simulink model "robotController"  (R2019b)
settings: Solver=FixedStepAuto  StartTime=0.0  StopTime=10.0  FixedStep=0.1  RelTol=1e-3
InitFcn:
  | set_param('robotController', 'ForceConsistencyChecking', 'off');
undefined symbols (not defined in the file): awayFromGoalThresh, loadingStation, logicalMap, unloadingStations
libraries: robotalgslib x1
settings Model: OrderedModelArguments=off  Creator=The MathWorks, Inc.  LastModifiedBy=Helsi
settings RTWCC: GenCodeOnly=on

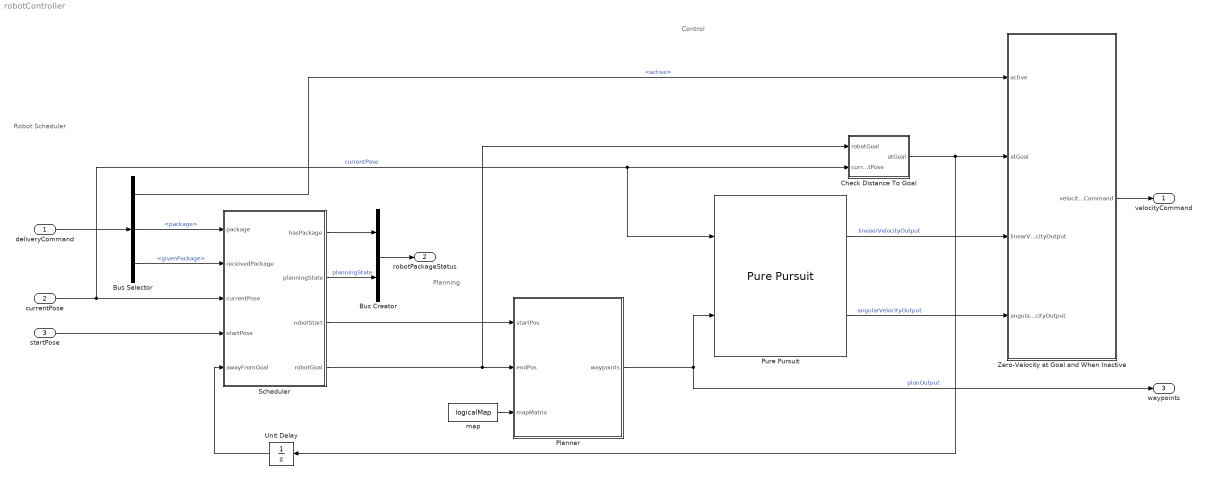
== system robotController ==
  note: Control
  note: Planning
  note: Robot Scheduler
  deliveryCommand : Inport  OutDataTypeStr=Bus: RobotDeliverCommand  BusOutputAsStruct=on
  currentPose : Inport  Port=2  PortDimensions=[3, 1]
  startPose : Inport  Port=3
  Bus Creator : BusCreator  Inputs=2  OutDataTypeStr=Bus: RobotPackageStatus  NonVirtualBus=on
      settings: InheritFromInputs=off
  Bus Selector : BusSelector  OutputSignals=active,package,givenPackage
  Check Distance To Goal : Subsystem
  Planner : MATLAB Function  TreatAsAtomicUnit=on
  Pure Pursuit : robotalgslib/Pure Pursuit  DesiredLinearVelocity=0.1  MaxAngularVelocity=1.0  LookaheadDistance=0.5  TargetDirPort=off  SimulateUsing=Code generation
      settings: SourceProductName=Navigation Toolbox  SourceProductBaseCode=NV
  Scheduler : Stateflow chart  Priority=2  BlockKeywords=__PRM__SERIALIZED__DATA__:Stateflow Chart,Stateflow Diagram
  Unit Delay : UnitDelay  SampleTime=-1  HasFrameUpgradeWarning=on
  Zero-Velocity at Goal and When Inactive : Subsystem
  map : Constant  Value=logicalMap
  velocityCommand : Outport
  robotPackageStatus : Outport  Port=2  OutDataTypeStr=Bus: RobotPackageStatus  BusOutputAsStruct=on
  waypoints : Outport  Port=3
  wires:
  Scheduler/2(planningState) -> Bus Creator/2  "planningState"
  Check Distance To Goal/1(atGoal) -> Unit Delay/1, Zero-Velocity at Goal and When Inactive/2(atGoal)
  Pure Pursuit/2 -> Zero-Velocity at Goal and When Inactive/4(angularVelocityOutput)  "angularVelocityOutput"
  Bus Selector/3 -> Scheduler/2(receivedPackage)  "<givenPackage>"
  Zero-Velocity at Goal and When Inactive/1(velocityCommand) -> velocityCommand/1
  currentPose/1 -> Pure Pursuit/1, Check Distance To Goal/2(currentPose), Scheduler/3(currentPose)  "currentPose"
  Bus Selector/1 -> Zero-Velocity at Goal and When Inactive/1(active)  "<active>"
  Unit Delay/1 -> Scheduler/5(awayFromGoal)
  Scheduler/1(hasPackage) -> Bus Creator/1
  Planner/1(waypoints) -> Pure Pursuit/2, waypoints/1  "planOutput"
  startPose/1 -> Scheduler/4(startPose)
  Bus Creator/1 -> robotPackageStatus/1
  map/1 -> Planner/3(mapMatrix)
  Scheduler/4(robotGoal) -> Planner/2(endPos), Check Distance To Goal/1(robotGoal)
  Pure Pursuit/1 -> Zero-Velocity at Goal and When Inactive/3(linearVelocityOutput)  "lineaerVelocityOutput"
  Bus Selector/2 -> Scheduler/1(package)  "<package>"
  deliveryCommand/1 -> Bus Selector/1
  Scheduler/3(robotStart) -> Planner/1(startPos)

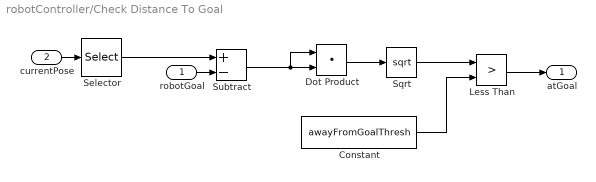
== system robotController/Check Distance To Goal ==
  robotGoal : Inport
  currentPose : Inport  Port=2
  Constant : Constant  Value=awayFromGoalThresh
  Dot Product : DotProduct  InputSameDT=on  OutDataTypeStr=Inherit: Inherit via internal rule
  Less Than : RelationalOperator  Operator=>  OutDataTypeStr=boolean  RndMeth=Simplest
  Selector : Selector  InputPortWidth=3  IndexOptions=Index vector (dialog)  Indices=[1 2]  OutputSizes=1
  Sqrt : Sqrt  SaturateOnIntegerOverflow=on
  Subtract : Sum  Inputs=+-
  atGoal : Outport
  wires:
  robotGoal/1 -> Subtract/2
  Dot Product/1 -> Sqrt/1
  Constant/1 -> Less Than/2
  currentPose/1 -> Selector/1
  Less Than/1 -> atGoal/1
  Sqrt/1 -> Less Than/1
  Subtract/1 -> Dot Product/1, Dot Product/2
  Selector/1 -> Subtract/1

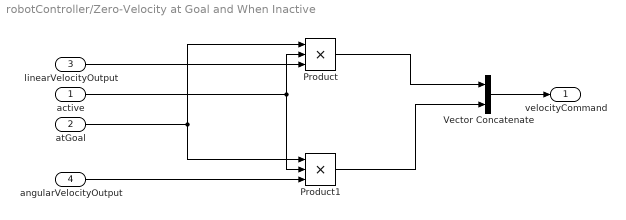
== system robotController/Zero-Velocity at Goal and When Inactive ==
  active : Inport
  atGoal : Inport  Port=2
  linearVelocityOutput : Inport  Port=3
  angularVelocityOutput : Inport  Port=4
  Product : Product  Inputs=3
  Product1 : Product  Inputs=3
  Vector Concatenate : Concatenate
  velocityCommand : Outport
  wires:
  active/1 -> Product/2, Product1/2
  Product/1 -> Vector Concatenate/1
  atGoal/1 -> Product/1, Product1/1
  Vector Concatenate/1 -> velocityCommand/1
  Product1/1 -> Vector Concatenate/2
  linearVelocityOutput/1 -> Product/3
  angularVelocityOutput/1 -> Product1/3

== matlab function robotController/Planner ==
  settings: updateMethod=DISCRETE
  data: startPos input size=[1 2]; endPos input size=[1 2]; waypoints output size=[100 2]; mapMatrix input
function waypoints = planning(startPos, endPos, mapMatrix)

persistent waypointsInternal
persistent prevStartPos
persistent prevEndPos

% Set constant parameters
maxNumNodes = 100;

% Initialize persistent variables that are used downstream
if isempty(prevStartPos)
    prevStartPos = startPos;
end

if isempty(prevEndPos)
    prevEndPos = endPos;
end

isNewPath = (~isequal(prevStartPos, startPos) || ~isequal(prevEndPos, endPos));

if isempty(waypointsInternal) || isNewPath
    % Two conditions in which waypoints must be set: they are not yet
    % initialized, or they are initialized, but the current start and end
    % do not match those used to generate the previous set of waypoints
    [waypointsInternal] = planPath(mapMatrix, maxNumNodes, startPos, endPos);
end

% Update the outputs
waypoints = waypointsInternal;

% Update the persistent variables that indicate previous state
prevStartPos = startPos;
prevEndPos = endPos;

%% Helper Function



end

function wayPoints = planPath(mapMatrix, maxNodes, startPos, endPos)
    
    % Create a probabilistic roadmap
    map = binaryOccupancyMap(mapMatrix);
    prm = mobileRobotPRM(map, maxNodes);
    
    % Find a path between two points
    xy = findpath(prm, startPos, endPos);
    wayPoints = repmat(endPos, maxNodes, 1);
    
    % Number of nodes that are actually used
    numNodes = length(xy);
    wayPoints(1:numNodes,:) = xy;    

end

== stateflow chart robotController/Scheduler ==
  settings: sampleTime=0.1
  state GoToUnloadingStation
    entry:
    robotGoal = unloadingStations(package, :)';
    robotStart = currentPose(1:2)';
  state GoToLoadingStation
    entry:
    robotGoal = loadingStation';
    robotStart = currentPose(1:2)';
  state StationHalt
    entry, during:
  (default) -> (junction 65) : {robotStart = startPose;
      | hasPackage = 0;
      | }
  (junction 65) -> GoToLoadingStation
  GoToLoadingStation -> StationHalt [order 1] : [hasPackage && package]
  StationHalt -> GoToUnloadingStation [order 1] : [planningState == RobotState.AtLoadingStn && ...
      | after(stopDelay, tick)]
  StationHalt -> GoToLoadingStation [order 2] : [planningState == RobotState.AtUnloadingStn && ...
      | after(stopDelay, tick)]
  GoToUnloadingStation -> StationHalt : [~awayFromGoal]
      | {planningState = RobotState.AtUnloadingStn;
      | hasPackage = 0;}
  GoToLoadingStation -> (junction 72) [order 2] : [~awayFromGoal]{planningState = RobotState.AtLoadingStn;}
  (junction 72) -> (junction 102) : [receivedPackage]{hasPackage = 1;}
  data: hasPackage output; planningState output Enum: RobotState =RobotState.AtDock; loadingStation parameter; robotStart output size=[1, 2]; robotGoal output size=2; unloadingStations parameter; package input; receivedPackage input; currentPose input; startPose input size=[1 2]; awayFromGoal input; stopDelay local =0.5e3
